simulink model "Angulo2"  (R2022a)
settings: Solver=FixedStepAuto  StartTime=0.0  StopTime=inf  FixedStep=0.01  RelTol=1e-3
model workspace (MAT data in the model file):
  Param = Simulink.Parameter
  Param.Value = 90
  Param.DataType = 'auto'
  Param.Complexity = 'real'
  Param.Dimensions = [1 1]
  SL_ROS_VariableLengthArrays_MaxSizes.CommonInfo.ArrayTruncateAction = 'EmitWarning'
  SL_ROS_VariableLengthArrays_MaxSizes.MsgTypeMap = containers.Map
  SL_ROS_VariableLengthArrays_MaxSizes.MsgTypeMap.serialization.keys = {'sensor_msgs/LaserScan'}
  SL_ROS_VariableLengthArrays_MaxSizes.MsgTypeMap.serialization.values{1}(1).PropertyName = 'intensities'
  SL_ROS_VariableLengthArrays_MaxSizes.MsgTypeMap.serialization.values{1}(1).DataType = 'single'
  SL_ROS_VariableLengthArrays_MaxSizes.MsgTypeMap.serialization.values{1}(1).MaxLength = 360
  SL_ROS_VariableLengthArrays_MaxSizes.MsgTypeMap.serialization.values{1}(2).PropertyName = 'ranges'
  SL_ROS_VariableLengthArrays_MaxSizes.MsgTypeMap.serialization.values{1}(2).DataType = 'single'
  SL_ROS_VariableLengthArrays_MaxSizes.MsgTypeMap.serialization.values{1}(2).MaxLength = 360
  SL_ROS_VariableLengthArrays_MaxSizes.MsgTypeMap.serialization.uniformity = 0
  SL_ROS_VariableLengthArrays_MaxSizes.MsgTypeMap.serialization.keyType = 'char'
  SL_ROS_VariableLengthArrays_MaxSizes.MsgTypeMap.serialization.valueType = 'any'
undefined symbols (not defined in the file): angular, header, linear, temperature
libraries: ros2lib x6, dspstat3 x2, simulink_extras x1
settings Model: Creator=Francisco  LastModifiedBy=Francisco
settings OptimizationCC: EnhancedBackFolding=on  PassReuseOutputArgsAs=Individual arguments  ZeroExternalMemoryAtStartup=off  ZeroInternalMemoryAtStartup=off  MaxStackSize=64  OptimizeBlockOrder=speed  DifferentSizesBufferReuse=on  EfficientTunableParamExpr=on
settings DebuggingCC: ParameterTunabilityLossMsg=error
settings SFSimCC: MATLABDynamicMemAlloc=off
settings RTWCC: SystemTargetFile=ert.tlc  HardwareBoard=Robot Operating System 2 (ROS 2)  TLCOptions="-aInlineSetEventsForThisBaseRateFcn=TLC_FALSE -aSuppressMultiTaskScheduler=TLC_FALSE  -aRateBasedStepFcn=0"  TemplateMakefile=ert_default_tmf  Toolchain=Colcon Tools  TargetLang=C++
settings CodeAppCC: ForceParamTrailComments=on  IgnoreCustomStorageClasses=off  OperatorAnnotations=on  SimulinkDataObjDesc=on  SFDataObjDesc=on  InsertBlockDesc=on
settings ERTTargetCC: CodeInterfacePackaging=C++ class  SupportContinuousTime=on  RootIOFormat=Structure reference

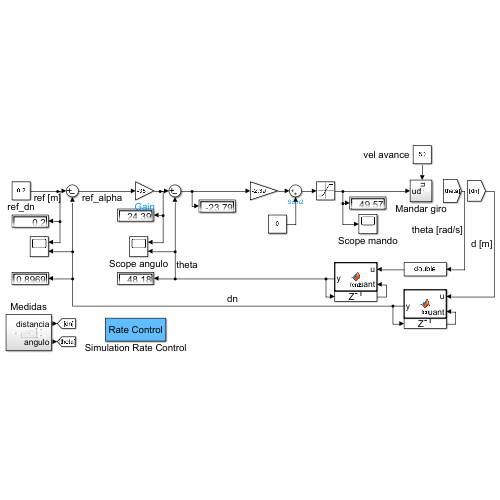
[thumbnail: Simulink's stored preview of the top-level diagram]
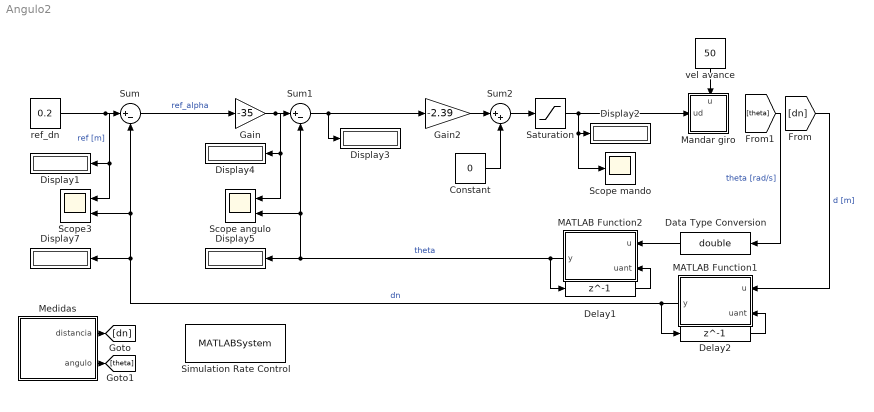
== system Angulo2 ==
  Constant : Constant  Value=0
  Data Type Conversion : DataTypeConversion  OutDataTypeStr=double  SaturateOnIntegerOverflow=off  RndMeth=Floor
  Delay1 : Delay  DelayLength=1
  Delay2 : Delay  DelayLength=1
  Display{1..5,7} (6 alike) : Display
  Gain : Gain  Gain=-35
  Gain2 : Gain  Gain=-2.39
  MATLAB Function1 : MATLAB Function  TreatAsAtomicUnit=on
  MATLAB Function2 : MATLAB Function  TreatAsAtomicUnit=on
  Mandar giro : Subsystem
      settings: PortSchema="{\"entries\":[{\"content\":{\"sides\":[{\"content\":{\"connectorIds\":[\"In1\"]},\"type\":\"ConnectorPlacement.EquallySpacedRectSide\",\"uuid\":\"62a47a31-29ea-4ff6-ada0-2f34531deb7e\"},{\"content\":{\"connectorIds\":[],\"side\":\"RIGHT\"},\"type\":\"ConnectorPlacement.EquallySpacedRectSide\",\"uuid\":\"cef9fc6f-4edd-47d5-b12f-7d71ad7c7192\"},{\"content\":{\"connectorIds\":[\"In2\"],\"side\":\"TOP\"},\"type\":\"ConnectorPlacement.EquallySpacedRectSide\",\"uuid\":\"d90855c6-0df1-43a0-b04e-b5b3218b95cf\"}]},\"type\":\"ConnectorPlacement.EquallySpacedConnector\",\"uuid\":\"9939f835-58b3-4645-8515-95471c9a01d3\"}],\"packageUris\":[\"http://schema.mathworks.com/mf0/Connector/R2020b\"],\"version\":\"1.0\"}"
  Medidas : Subsystem
  Saturation : Saturate  UpperLimit=50  LowerLimit=-50  LinearizeAsGain=off
  Scope angulo : Scope  NumInputPorts=2
  Scope mando : Scope
  Scope3 : Scope  NumInputPorts=2
  Simulation Rate Control : MATLABSystem  System=ExampleHelperSimulationRateControl  SampleTime=0.01
      mask Type: ExampleHelperSimulationRateControl
      mask Display: disp('Rate Control');
  Sum : Sum  Inputs=|+-
  Sum1 : Sum  Inputs=|+-
  Sum2 : Sum  Inputs=|++
  ref_dn : Constant  Value=0.2
  vel avance : Constant  Value=50
  wires:
  Sum/1 -> Gain/1  "ref_alpha"
  [dn] -> MATLAB Function1/1(u)  "d [m]"
  Medidas/1(distancia) -> [dn]
  Medidas/2(angulo) -> [theta]
  Gain2/1 -> Sum2/1
  MATLAB Function1/1(y) -> Display7/1, Scope3/2, Sum/2, Delay2/1  "dn"
  vel avance/1 -> Mandar giro/2(u)
  Delay2/1 -> MATLAB Function1/2(uant)
  Delay1/1 -> MATLAB Function2/2(uant)
  [theta] -> Data Type Conversion/1  "theta [rad/s]"
  Data Type Conversion/1 -> MATLAB Function2/1(u)
  Saturation/1 -> Display2/1, Scope mando/1, Mandar giro/1(ud)
  Sum1/1 -> Gain2/1, Display3/1
  MATLAB Function2/1(y) -> Sum1/2, Scope angulo/2, Display5/1, Delay1/1  "theta"
  Gain/1 -> Scope angulo/1, Display4/1, Sum1/1
  ref_dn/1 -> Sum/1, Scope3/1, Display1/1  "ref [m]"
  Sum2/1 -> Saturation/1
  Constant/1 -> Sum2/2

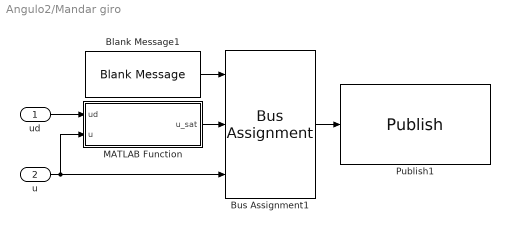
== system Angulo2/Mandar giro ==
  ud : Inport
  u : Inport  Port=2
  Blank Message1 : ros2lib/Blank Message  messageClass=Message  entityType=geometry_msgs/Twist  messageType=geometry_msgs/Twist  SampleTime=inf
      settings: SourceProductBaseCode=RR
  Bus Assignment1 : BusAssignment  AssignedSignals=angular.z,linear.x
  MATLAB Function : MATLAB Function  TreatAsAtomicUnit=on
  Publish1 : ros2lib/Publish  topicSource=Select from ROS network  topic=/cmd_vel  messageType=geometry_msgs/Twist  QOSHistory=Keep last  QOSDepth=1  QOSReliability=Reliable  QOSDurability=Volatile
      settings: SourceProductBaseCode=RR
  wires:
  Bus Assignment1/1 -> Publish1/1
  Blank Message1/1 -> Bus Assignment1/1
  u/1 -> MATLAB Function/2(u), Bus Assignment1/3
  MATLAB Function/1(u_sat) -> Bus Assignment1/2
  ud/1 -> MATLAB Function/1(ud)

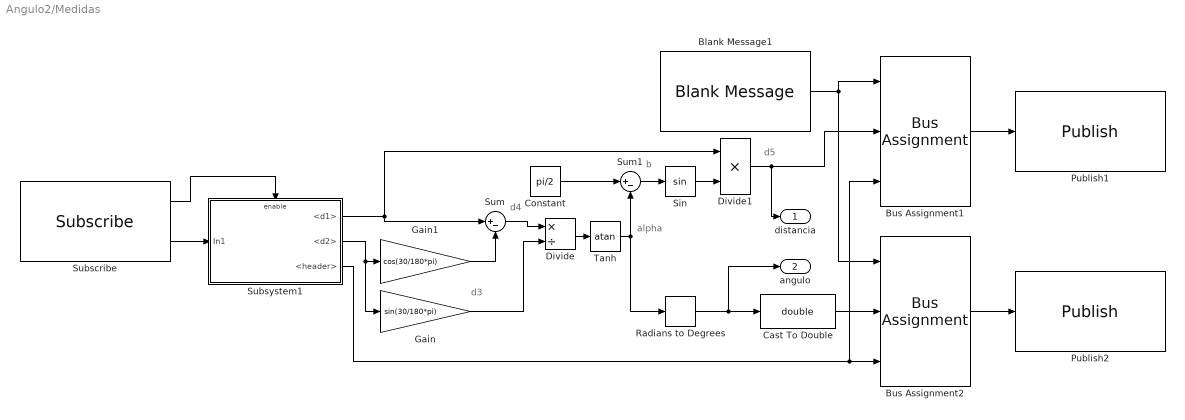
== system Angulo2/Medidas ==
  note: d5
  note: b
  note: alpha
  note: d3
  note: d4
  Blank Message1 : ros2lib/Blank Message  messageClass=Message  entityType=sensor_msgs/Temperature  messageType=sensor_msgs/Temperature  SampleTime=-1
      settings: SourceProductBaseCode=RR
  Bus Assignment1 : BusAssignment  AssignedSignals=temperature,header
  Bus Assignment2 : BusAssignment  AssignedSignals=temperature,header
  Cast To Double : DataTypeConversion  OutDataTypeStr=double  SaturateOnIntegerOverflow=off  RndMeth=Floor
  Constant : Constant  Value=pi/2
  Divide : Product  Inputs=*/
  Divide1 : Product  Inputs=**
  Gain : Gain  Gain=sin(30/180*pi)
  Gain1 : Gain  Gain=cos(30/180*pi)
  Publish1 : ros2lib/Publish  topicSource=Specify your own  topic=/distanciaPared  messageType=sensor_msgs/Temperature  QOSHistory=Keep last  QOSDepth=1  QOSReliability=Reliable  QOSDurability=Volatile
      settings: SourceProductBaseCode=RR
  Publish2 : ros2lib/Publish  topicSource=Specify your own  topic=/anguloPared  messageType=sensor_msgs/Temperature  QOSHistory=Keep last  QOSDepth=1  QOSReliability=Reliable  QOSDurability=Volatile
      settings: SourceProductBaseCode=RR
  Radians to Degrees : simulink_extras/Transformations/Radians to Degrees
  Sin : Trigonometry
  Subscribe : ros2lib/Subscribe  topicSource=Select from ROS network  topic=/scan  messageType=sensor_msgs/LaserScan  sampleTime=-1  QOSHistory=Keep last  QOSDepth=10  QOSReliability=Best effort  QOSDurability=Volatile
      settings: SourceProductBaseCode=RR
  Subsystem1 : Subsystem
  Sum : Sum  Inputs=|+-
  Sum1 : Sum  Inputs=|+-
  Tanh : Trigonometry  Operator=atan
  distancia : Outport
  angulo : Outport  Port=2
  wires:
  Subscribe/1 -> Subsystem1/Enable
  Constant/1 -> Sum1/1
  Subsystem1/1(<d1>) -> Sum/1, Divide1/1
  Subsystem1/2(<d2>) -> Gain/1, Gain1/1
  Subscribe/2 -> Subsystem1/1(In1)
  Cast To Double/1 -> Bus Assignment2/2
  Gain/1 -> Divide/2
  Sum/1 -> Divide/1
  Gain1/1 -> Sum/2
  Sin/1 -> Divide1/2
  Tanh/1 -> Sum1/2, Radians to Degrees/1
  Divide/1 -> Tanh/1
  Radians to Degrees/1 -> angulo/1, Cast To Double/1
  Subsystem1/3(<header>) -> Bus Assignment1/3, Bus Assignment2/3
  Sum1/1 -> Sin/1
  Bus Assignment1/1 -> Publish1/1
  Bus Assignment2/1 -> Publish2/1
  Blank Message1/1 -> Bus Assignment2/1, Bus Assignment1/1
  Divide1/1 -> distancia/1, Bus Assignment1/2

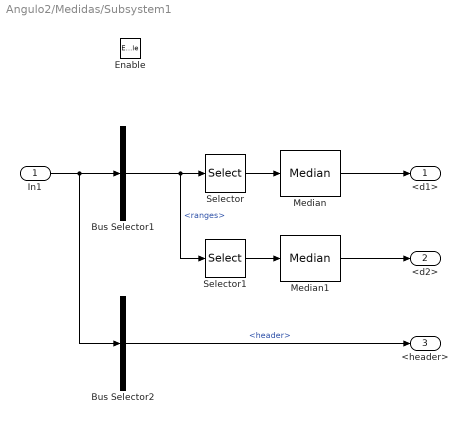
== system Angulo2/Medidas/Subsystem1 ==
  In1 : Inport
  Enable : EnablePort
  Bus Selector1 : BusSelector  OutputSignals=ranges
  Bus Selector2 : BusSelector  OutputSignals=header
  Median : dspstat3/Median  sortAlg=Quick sort  directionMode=Each column  dimension=1  roundingMode=Floor  overflowMode=off  accumDataTypeStr=Inherit: Same as product output  accumLastDataTypeStr=Inherit: Same as product output  outputDataTypeStr=Inherit: Same as accumulator  outputMin=[]  outputMax=[]  outputLastDataTypeStr=Inherit: Same as accumulator
      settings: SourceProductBaseCode=DS  allowOverrides=off
  Median1 : dspstat3/Median  sortAlg=Quick sort  directionMode=Each column  dimension=1  roundingMode=Floor  overflowMode=off  accumDataTypeStr=Inherit: Same as product output  accumLastDataTypeStr=Inherit: Same as product output  outputDataTypeStr=Inherit: Same as accumulator  outputMin=[]  outputMax=[]  outputLastDataTypeStr=Inherit: Same as accumulator
      settings: SourceProductBaseCode=DS  allowOverrides=off
  Selector : Selector  IndexMode=Zero-based  InputPortWidth=360  IndexOptions=Index vector (dialog)  Indices=[88:92]  OutputSizes=1
  Selector1 : Selector  IndexMode=Zero-based  InputPortWidth=360  IndexOptions=Index vector (dialog)  Indices=[118:122]  OutputSizes=1
  <d1> : Outport
  <d2> : Outport  Port=2
  <header> : Outport  Port=3
  wires:
  In1/1 -> Bus Selector2/1, Bus Selector1/1
  Bus Selector1/1 -> Selector1/1, Selector/1  "<ranges>"
  Selector/1 -> Median/1
  Selector1/1 -> Median1/1
  Median/1 -> <d1>/1
  Median1/1 -> <d2>/1
  Bus Selector2/1 -> <header>/1  "<header>"

== matlab function Angulo2/MATLAB Function2 ==
  data: u input; y output; uant input
function y = fcn2(u,uant)
if (abs(u)>= 58)
    y=uant;
else
    y=u;
end
end

== matlab function Angulo2/Mandar giro/MATLAB Function ==
  data: ud input; u input; u_sat output
function u_sat = LIMIT_MOTOR(ud,u)

if(abs(ud+u)>100)
  u_sat = u-100;
elseif(abs(-ud+u)>100)
  u_sat = -u-100;
else
  u_sat = ud  ;
end

end

== matlab function Angulo2/MATLAB Function1 ==
  data: u input; y output; uant input
function y = fcn(u,uant)
    if (u<= 0.001)
        y=uant;
    else
        y=u;
    end
end
